simulink model "practika2"  (R2024a)
settings: Solver=VariableStepAuto  StartTime=0.0  StopTime=15  RelTol=1e-3
model workspace (MAT data in the model file):
  b = 0.3
  diff_x = 0
  g = 9.81
  int_x = 0
  l = 0.5
  m = 0.5
  x = [1; 0]
  x1 = [-5; 0]
settings Model: Creator=Кирилл  LastModifiedBy=Анастасия
settings OptimizationCC: ReuseModelBlockBuffer=off
settings RTWCC: GPUComputeCapability=3.5

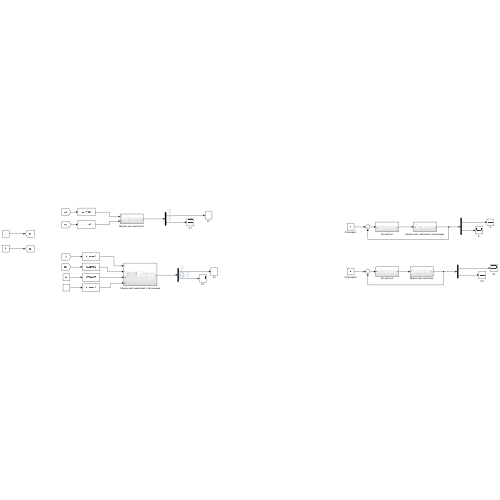
[thumbnail: Simulink's stored preview of the top-level diagram]
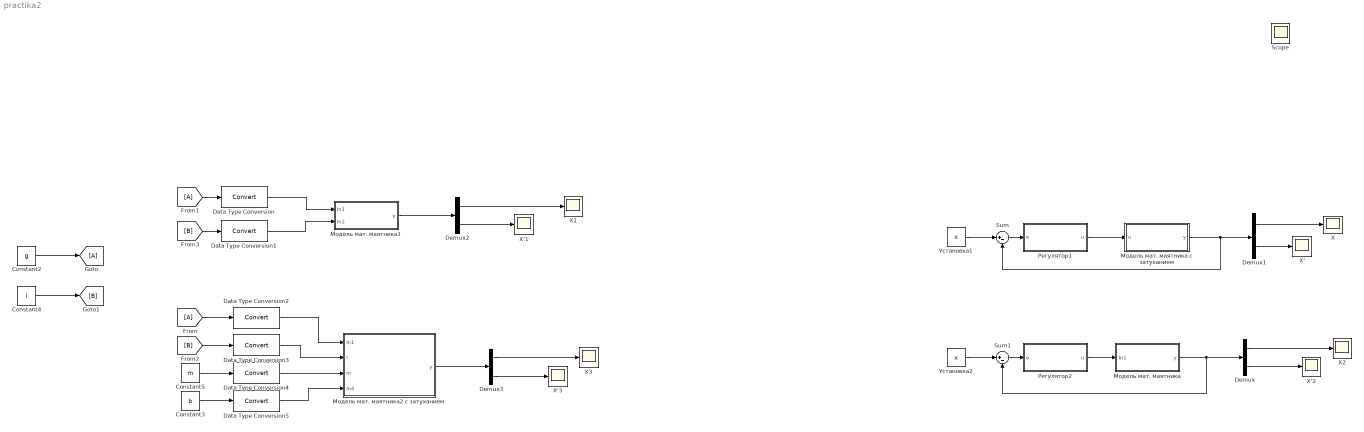
== system practika2 ==
  Constant2 : Constant  Value=g
  Constant3 : Constant  Value=b
  Constant4 : Constant  Value=l
  Constant5 : Constant  Value=m
  Data Type Conversion{,1..5} (6 alike) : DataTypeConversion  SaturateOnIntegerOverflow=off  RndMeth=Floor
  Demux{,1..3} (4 alike) : Demux  Outputs=2
  From : From
  From1 : From
  Goto : Goto
  Sum : Sum  Inputs=|+-
  Sum1 : Sum  Inputs=|+-
  X{,1..3} (4 alike) : Scope
  X'{,1..3} (4 alike) : Scope
  Модель мат. маятника : Subsystem
  "Модель мат. маятника c затуханием " : Subsystem
  Модель мат. маятника1 : Subsystem
  Модель мат. маятника2 c затуханием : Subsystem
  Регулятор1 : Subsystem
  Регулятор2 : Subsystem
  Установка1 : Constant  Value=x
  Установка2 : Constant  Value=x
  Scope : Scope
  wires:
  Установка1/1 -> Sum/1
  "Модель мат. маятника c затуханием "/1(y) -> Sum/2, Demux1/1
  Sum/1 -> Регулятор1/1(e)
  Регулятор1/1(u) -> "Модель мат. маятника c затуханием "/1(u)
  Demux1/1 -> X/1
  Demux1/2 -> X'/1
  Установка2/1 -> Sum1/1
  Sum1/1 -> Регулятор2/1(e)
  Регулятор2/1(u) -> Модель мат. маятника/1(In1)
  Модель мат. маятника/1(y) -> Sum1/2, Demux/1
  Demux/1 -> X2/1
  Demux/2 -> X'2/1
  From1/1 -> Data Type Conversion/1
  [B] -> Data Type Conversion1/1
  Модель мат. маятника1/1(y) -> Demux2/1
  Demux2/2 -> X'1/1
  Demux2/1 -> X1/1
  Модель мат. маятника2 c затуханием/1(y) -> Demux3/1
  Demux3/2 -> X'3/1
  Demux3/1 -> X3/1
  Constant5/1 -> Data Type Conversion4/1
  Constant3/1 -> Data Type Conversion5/1
  Data Type Conversion/1 -> Модель мат. маятника1/1(In1)
  Data Type Conversion1/1 -> Модель мат. маятника1/2(In2)
  Data Type Conversion5/1 -> Модель мат. маятника2 c затуханием/4(In4)
  Data Type Conversion4/1 -> Модель мат. маятника2 c затуханием/3(m)
  Data Type Conversion3/1 -> Модель мат. маятника2 c затуханием/2(l)
  Data Type Conversion2/1 -> Модель мат. маятника2 c затуханием/1(In1)
  Constant2/1 -> Goto/1
  From/1 -> Data Type Conversion2/1
  Constant4/1 -> [B]
  [B] -> Data Type Conversion3/1

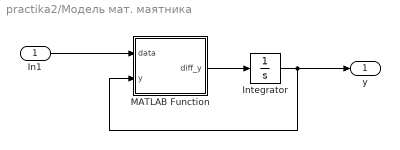
== system practika2/Модель мат. маятника ==
  In1 : Inport
  Integrator : Integrator  InitialCondition=x1
  MATLAB Function : MATLAB Function  TreatAsAtomicUnit=on
  y : Outport
  wires:
  MATLAB Function/1(diff_y) -> Integrator/1
  Integrator/1 -> y/1, MATLAB Function/2(y)
  In1/1 -> MATLAB Function/1(data)

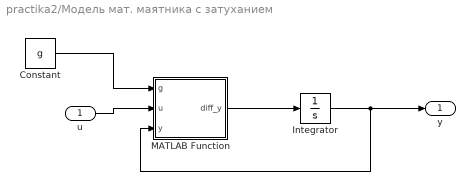
== system practika2/Модель мат. маятника c затуханием  ==
  u : Inport
  Constant : Constant  Value=g
  Integrator : Integrator  InitialCondition=[-2;0]
  MATLAB Function : MATLAB Function  TreatAsAtomicUnit=on
  y : Outport
  wires:
  MATLAB Function/1(diff_y) -> Integrator/1
  Integrator/1 -> MATLAB Function/3(y), y/1
  u/1 -> MATLAB Function/2(u)
  Constant/1 -> MATLAB Function/1(g)

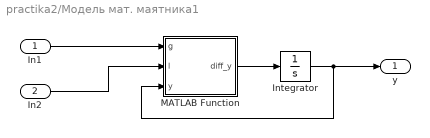
== system practika2/Модель мат. маятника1 ==
  In1 : Inport
  In2 : Inport  Port=2
  Integrator : Integrator  InitialCondition=x1
  MATLAB Function : MATLAB Function  TreatAsAtomicUnit=on
  y : Outport
  wires:
  MATLAB Function/1(diff_y) -> Integrator/1
  Integrator/1 -> MATLAB Function/3(y), y/1
  In1/1 -> MATLAB Function/1(g)
  In2/1 -> MATLAB Function/2(l)

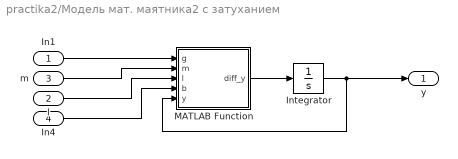
== system practika2/Модель мат. маятника2 c затуханием ==
  In1 : Inport
  l : Inport  Port=2
  m : Inport  Port=3
  In4 : Inport  Port=4
  Integrator : Integrator  InitialCondition=x1
  MATLAB Function : MATLAB Function  TreatAsAtomicUnit=on
  y : Outport
  wires:
  MATLAB Function/1(diff_y) -> Integrator/1
  Integrator/1 -> y/1, MATLAB Function/5(y)
  In1/1 -> MATLAB Function/1(g)
  l/1 -> MATLAB Function/3(l)
  m/1 -> MATLAB Function/2(m)
  In4/1 -> MATLAB Function/4(b)

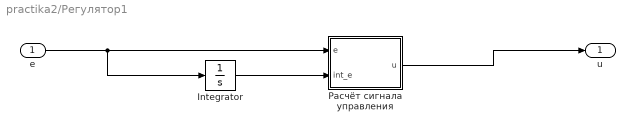
== system practika2/Регулятор1 ==
  e : Inport
  Integrator : Integrator
  Расчёт сигнала управления : MATLAB Function  TreatAsAtomicUnit=on
  u : Outport
  wires:
  e/1 -> Расчёт сигнала управления/1(e), Integrator/1
  Integrator/1 -> Расчёт сигнала управления/2(int_e)
  Расчёт сигнала управления/1(u) -> u/1

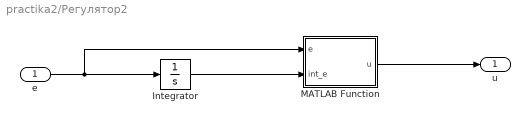
== system practika2/Регулятор2 ==
  e : Inport
  Integrator : Integrator
  MATLAB Function : MATLAB Function  TreatAsAtomicUnit=on
  u : Outport
  wires:
  e/1 -> MATLAB Function/1(e), Integrator/1
  Integrator/1 -> MATLAB Function/2(int_e)
  MATLAB Function/1(u) -> u/1

== matlab function practika2/Модель мат. маятника c затуханием /MATLAB Function ==
  data: g input; u input; diff_y output; y input
function diff_y = fcn(g, u, y)

l = 1;
m = 1;
b = 1;

%diff_y=[y(2); -(g/l)*sin(y(1)) - (b*y(2))/(m*(l^2)) - c*y(1)/(m*(l^2))+ u/(m*(l^2)) ];
diff_y=[y(2); -(g/l)*sin(y(1)) - (b*y(2))/(m)];

end

== matlab function practika2/Регулятор1/Расчёт сигнала управления ==
  data: e input; int_e input; u output
function u = fcn(e, int_e)
Kp = 2;
K1 = 2;


u = Kp*e(1) + Kp*e(2) + K1*int_e(1) + K1*int_e(2);
end

== matlab function practika2/Модель мат. маятника/MATLAB Function ==
  data: data input; diff_y output; y input
function diff_y = fcn(data, y)

    g = 9.81;
    l = 0.1;
    m = 0.5;

    % diff_y(1, 2) = -(g/l)*sin(y(1)) - (b*y(2))/(m*(l^2)) - c*y(1)/(m*(l^2)) + u/(m*(l^2));

    diff_y=[y(2); -(g/l)*sin(y(1))];

end

== matlab function practika2/Регулятор2/MATLAB Function ==
  data: e input; int_e input; u output
function u = fcn(e, int_e)

    K1 = 2;
    K2 = 0.5;
    
    u=K1*e(1)+K1*e(2)+K2*int_e(1)+K2*int_e(2);
    
end

== matlab function practika2/Модель мат. маятника1/MATLAB Function ==
  data: g input; l input; y input; diff_y output
function diff_y = fcn(g, l, y)


    % diff_y(1, 2) = -(g/l)*sin(y(1)) - (b*y(2))/(m*(l^2)) - c*y(1)/(m*(l^2)) + u/(m*(l^2));

    diff_y=[y(2); -(g/l)*sin(y(1))];

end

== matlab function practika2/Модель мат. маятника2 c затуханием/MATLAB Function ==
  data: g input; m input; l input; b input; y input; diff_y output
function diff_y = fcn(g, m, l, b, y)

    diff_y=[y(2); -(g/l)*sin(y(1)) - (b*y(2))/(m)];
end
